simulink model "test3_HSV"  (R2020b)
settings: Solver=ode4  StartTime=0.0  StopTime=60  RelTol=1e-3
undefined symbols (not defined in the file or in its folder): gray, none, videoinput
libraries: dspvision x2, visionsources x2, imaqlib x1
settings Model: Creator=Amir  LastModifiedBy=vahed
settings DataIOCC: ReturnWorkspaceOutputs=off
settings DebuggingCC: ArithmeticOperatorsInVariantConditions=warning
settings SFSimCC: CustomCodeUndefinedFunction=UseInterfaceOnly
settings RTWCC: Description=Simulink Desktop Real-Time  SystemTargetFile=sldrt.tlc  TemplateMakefile=sldrt.tmf  RTWCompilerOptimization=on
settings CodeAppCC: MaxIdLength=95
settings SimulinkDesktopRealTimeCC: TargetPreCompLibLocation=C:\Program Files\Polyspace\R2020b\toolbox\sldrt\lib\win64

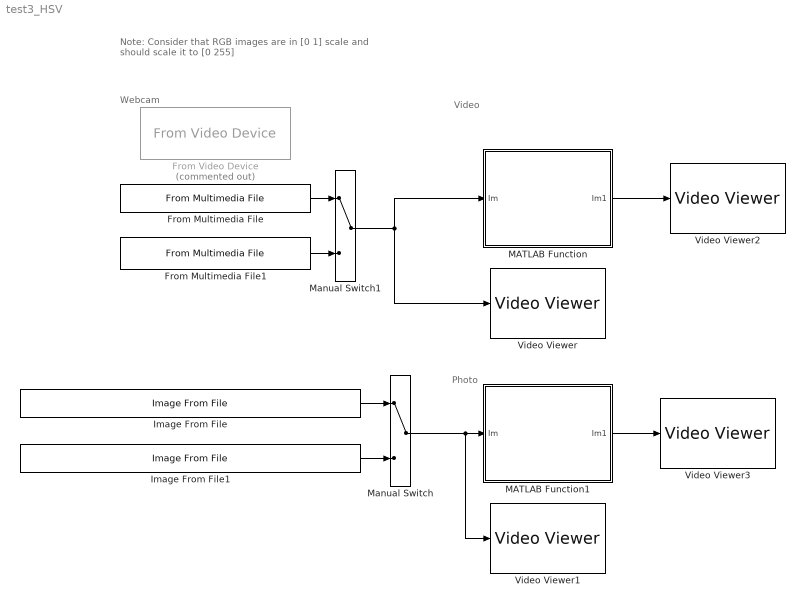
== system test3_HSV ==
  note: Webcam
  note: Photo
  note: Note:
      | Consider that RGB images are in [0 1] scale and should
      | scale it to [0 255]
  note: Video
  From Multimedia File : dspvision/From Multimedia File  inputFilename=Forest_Fire_Stream.wmv  readRange=[1 Inf]  loop=on  numPlays=inf  outputStreams=Video only  videoDataType=single  audioDataType=double  inheritSampleTime=on  userDefinedSampleTime=1/30  noAudioOutput=off  isIntensityVideo=off  fourcc=RGB  colorVideoFormat=One multidimensional signal  outputEOF=off  dataOrg=Column-major  audioFrameSize=1024  computeAudioFrameSize=off  outSamplingMode=Sample based
  From Multimedia File1 : dspvision/From Multimedia File  inputFilename=Controlled_Burn_Stream.wmv  readRange=[1 Inf]  loop=on  numPlays=inf  outputStreams=Video only  videoDataType=single  audioDataType=double  inheritSampleTime=on  userDefinedSampleTime=1/30  noAudioOutput=off  isIntensityVideo=off  fourcc=RGB  colorVideoFormat=One multidimensional signal  outputEOF=off  dataOrg=Column-major  audioFrameSize=1024  computeAudioFrameSize=off  outSamplingMode=Sample based
  From Video Device : imaqlib/From Video Device  Commented=on  DeviceMenu=(none)  Device=winvideo 1 (USB2.0 HD UVC WebCam)  ObjConstructor=videoinput('winvideo', 1)  VideoFormatMenu=(none)  VideoFormat=MJPG_640x480  VideoSource=input1  ROIPosition=[0 0 480 640]  EnableHWTrigger=off  TriggerConfiguration=none/none  SampleTime=0.001  OutputPortsMode=One multidimensional signal  DataType=double  CanDoHWTrigger=no  ReturnedColorSpace=rgb  BlockHandle=17.0001  ROIWidth=640  ROIHeight=480  ROIColumn=0  ROIRow=0  EngXMLPath=C:\Program Files\Polyspace\R2020b\toolbox\imaq\imaq\private  DevXMLPath=C:\ProgramData\MATLAB\SupportPackages\R2018b\toolbox\imaq\supportpackages\genericvideo\adaptor\win64  EngLibPath=C:\Program Files\Polyspace\R2020b\toolbox\imaq\imaqblks\imaqmex\win64  ColorSpace=rgb  BayerSensorAlignment=grbg  ImaqMode=off
  Image From File : visionsources/Image From File  Tag=vipblks_nd  FileName=growing-risk-future-wildfires_adobestock_199370851.jpeg  Ts=inf  imagePorts=One multidimensional signal  OutPortLabels=R|G|B  ImageDataType=Inherit from input image  sdImageDataType=uint(8)  Signed=on  WordLength=16  FractionLengthMode=User-defined  FractionLength=15
  Image From File1 : visionsources/Image From File  Tag=vipblks_nd  FileName=fotolia-gilitukha-forest-fire.jpg  Ts=inf  imagePorts=One multidimensional signal  OutPortLabels=R|G|B  ImageDataType=Inherit from input image  sdImageDataType=uint(8)  Signed=on  WordLength=16  FractionLengthMode=User-defined  FractionLength=15
  MATLAB Function : MATLAB Function  TreatAsAtomicUnit=on
  MATLAB Function1 : MATLAB Function  TreatAsAtomicUnit=on
  Manual Switch : ManualSwitch
  Manual Switch1 : ManualSwitch
  Video Viewer : VideoViewer  colormapValue=gray(256)  FigPos=[43.6666666666667 648 674.666666666667 508.666666666667]
  Video Viewer1 : VideoViewer  colormapValue=gray(256)  FigPos=[233.666666666667 1007.33333333333 674.666666666667 508.666666666667]
  Video Viewer2 : VideoViewer  colormapValue=gray(256)  FigPos=[767 685.333333333333 675.333333333333 509.333333333333]
  Video Viewer3 : VideoViewer  colormapValue=gray(256)  FigPos=[939 1058 675.333333333333 509.333333333333]
  wires:
  Manual Switch1/1 -> MATLAB Function/1(Im), Video Viewer/1
  MATLAB Function/1(Im1) -> Video Viewer2/1
  MATLAB Function1/1(Im1) -> Video Viewer3/1
  Image From File/1 -> Manual Switch/1
  Image From File1/1 -> Manual Switch/2
  Manual Switch/1 -> Video Viewer1/1, MATLAB Function1/1(Im)
  From Multimedia File/1 -> Manual Switch1/1
  From Multimedia File1/1 -> Manual Switch1/2

== matlab function test3_HSV/MATLAB Function1 ==
  data: Im input; Im1 output
function Im1 = fcn(Im)
Im=Im;
% .*255;
[m,n,~]=size(Im);
mask=zeros(m,n);
Im_HSV = rgb2hsv(Im);
R_T=115;%[115 135]
S_T=55;%[55 65]
for i=1:m
    for j=1:n
        if Im(i,j,1)>=R_T
            if Im(i,j,1)>=Im(i,j,2) && Im(i,j,2)>=Im(i,j,3)
                if Im_HSV(i,j,2)>=(255-Im(i,j,1))*S_T/R_T
                    mask(i,j)=1;
                end
            end
        end
    end
end
Im1= bsxfun(@times, Im, cast(mask, 'like', Im));
% ./255;
% [y,x]=find(mask);
% x_min=1;y_min=1;x_max=1;y_max=1;
% if ~isempty(x)
%     x_min=10000;y_min=10000;x_max=1;y_max=1;
%     for i=1:length(x)
%         for j=1:length(x)
%             if mask(y(i),x(j))==1
%                 if i<x_min
%                     x_min=i;
% %                 end
% %                 if j<y_min
%                     y_min=j;
%                 end
%                 if i>x_max
%                     x_max=i;
% %                 end
% %                 if j<y_max
%                     y_max=j;
%                 end
%             end
%         end
%     end
% end
% pts=[x_min y_min (x_max-x_min) (y_max-y_min)];

== matlab function test3_HSV/MATLAB Function ==
  data: Im input; Im1 output
function Im1 = fcn(Im)
Im=Im.*255;
[m,n,~]=size(Im);
mask=zeros(m,n);
Im_HSV = rgb2hsv(Im);
R_T=115;%[115 135]
S_T=55;%[55 65]
for i=1:m
    for j=1:n
        if Im(i,j,1)>=R_T
            if Im(i,j,1)>=Im(i,j,2) && Im(i,j,2)>=Im(i,j,3)
                if Im_HSV(i,j,2)>=(255-Im(i,j,1))*S_T/R_T
                    mask(i,j)=1;
                end
            end
        end
    end
end
Im1= bsxfun(@times, Im, cast(mask, 'like', Im))./255;
% [y,x]=find(mask);
% x_min=1;y_min=1;x_max=1;y_max=1;
% if ~isempty(x)
%     x_min=10000;y_min=10000;x_max=1;y_max=1;
%     for i=1:length(x)
%         for j=1:length(x)
%             if mask(y(i),x(j))==1
%                 if i<x_min
%                     x_min=i;
% %                 end
% %                 if j<y_min
%                     y_min=j;
%                 end
%                 if i>x_max
%                     x_max=i;
% %                 end
% %                 if j<y_max
%                     y_max=j;
%                 end
%             end
%         end
%     end
% end
% pts=[x_min y_min (x_max-x_min) (y_max-y_min)];
